simulink model "hw_reuse"  (R2018a)
settings: Solver=FixedStepDiscrete  StartTime=0.0  StopTime=1000*ts  RelTol=1e-3
libraries: simulink x1
settings Model: DataTypeOverride=Off  Creator=CIDEI  LastModifiedBy=pcoss
settings DataIOCC: SaveOutput=off  SaveTime=off
settings OptimizationCC: BlockReduction=off  ConditionallyExecuteInputs=off  DefaultParameterBehavior=Inlined  LifeSpan=inf
settings DebuggingCC: AlgebraicLoopMsg=error  SingleTaskRateTransMsg=error  StrictBusMsg=ErrorOnBusTreatedAsVector  SFUnexpectedBacktrackingDiag=warning  SFNoUnconditionalDefaultTransitionDiag=warning  SFExecutionAtInitializationDiag=none
settings HardwareCC: ProdBitPerPointer=32  ProdBitPerSizeT=32  ProdBitPerPtrDiffT=32  ProdLargestAtomicFloat=None  ProdIntDivRoundTo=Undefined  ProdEndianess=Unspecified  ProdWordSize=32  ProdHWDeviceType=ASIC/FPGA->ASIC/FPGA  ProdEqTarget=off
settings CodeAppCC: StateflowObjectComments=on
settings GRTTargetCC: TargetLangStandard=C89/C90 (ANSI)
settings ConfigComp: CovMetricSettings=dw  CovHtmlReporting=on  CovSaveCumulativeToWorkspaceVar=on  CovSaveSingleToWorkspaceVar=on  CovExternalEMLEnable=off

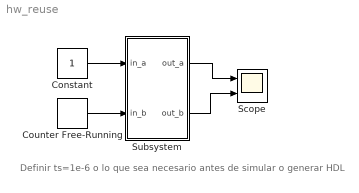
== system hw_reuse ==
  note: Definir ts=1e-6 o lo que sea necesario antes de simular o generar HDL
  Constant : Constant  OutDataTypeStr=fixdt(1,8,0)  SampleTime=-1
  Counter Free-Running : simulink/Sources/Counter Free-Running  NumBits=8  tsamp=ts
  Scope : Scope  NumInputPorts=2
  Subsystem : Subsystem
  wires:
  Constant/1 -> Subsystem/1(in_a)
  Counter Free-Running/1 -> Subsystem/2(in_b)
  Subsystem/1(out_a) -> Scope/1
  Subsystem/2(out_b) -> Scope/2

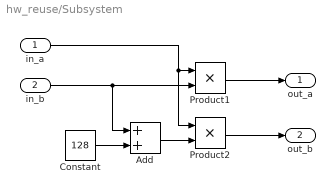
== system hw_reuse/Subsystem ==
  in_a : Inport
  in_b : Inport  Port=2
  Add : Sum  OutDataTypeStr=Inherit: Same as accumulator
  Constant : Constant  Value=128  OutDataTypeStr=fixdt(0,8,0)  SampleTime=-1
  Product1 : Product
  Product2 : Product
  out_a : Outport
  out_b : Outport  Port=2
  wires:
  Product2/1 -> out_b/1
  Constant/1 -> Add/2
  Add/1 -> Product2/2
  in_a/1 -> Product2/1, Product1/1
  in_b/1 -> Add/1, Product1/2
  Product1/1 -> out_a/1
